simulink model "udpConnector"  (R2018b)
settings: Solver=VariableStepAuto  StartTime=0.0  StopTime=1000  RelTol=1e-3
undefined symbols (not defined in the file): f
libraries: instrumentlib x2
settings Model: Creator=root  LastModifiedBy=yuto

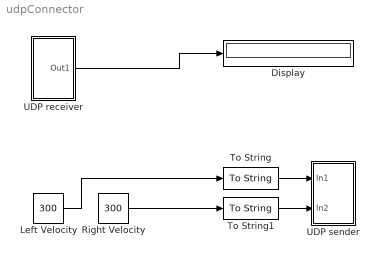
== system udpConnector ==
  Display : Display
  "Left Velocity " : Constant  Value=300
  Right Velocity : Constant  Value=300
  To String : ToString
  To String1 : ToString
  UDP receiver : Subsystem
  "UDP sender " : Subsystem
  wires:
  "Left Velocity "/1 -> To String/1
  UDP receiver/1(Out1) -> Display/1
  To String/1 -> "UDP sender "/1(In1)
  To String1/1 -> "UDP sender "/2(In2)
  Right Velocity/1 -> To String1/1

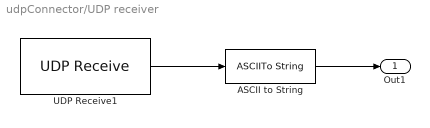
== system udpConnector/UDP receiver ==
  ASCII to String : ASCIIToString
  UDP Receive1 : instrumentlib/UDP Receive  Host=localhost  Port=9090  LocalPort=50002  EnablePortSharing=off  GetLatestData=off  DataSize="[23   1]"  DataType=uint8  ASCIIFormatting=%f,  Terminator=LF  ByteOrder=BigEndian  EnableBlockingMode=on  Timeout=10  SampleTime=0.01  LocalAddress=localhost
      settings: SourceProductName=Instrument Control Toolbox
  Out1 : Outport
  wires:
  UDP Receive1/1 -> ASCII to String/1
  ASCII to String/1 -> Out1/1

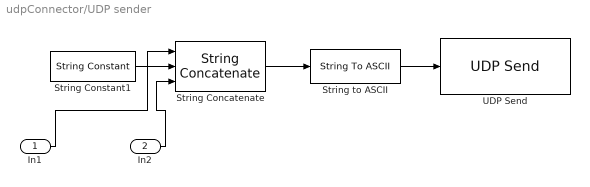
== system udpConnector/UDP sender  ==
  In1 : Inport
  In2 : Inport  Port=2
  String Concatenate : StringConcatenate  Inputs=3
  String Constant1 : StringConstant  String="\",\""
  String to ASCII : StringToASCII
  UDP Send : instrumentlib/UDP Send  Host=localhost  Port=50003  LocalPort=-1  EnablePortSharing=off  ByteOrder=BigEndian  OutputDatagramPacketSize=512  EnableBlockingMode=on  LocalAddress=0.0.0.0
      settings: SourceProductName=Instrument Control Toolbox
  wires:
  In2/1 -> String Concatenate/3
  In1/1 -> String Concatenate/1
  String Concatenate/1 -> String to ASCII/1
  String to ASCII/1 -> UDP Send/1
  String Constant1/1 -> String Concatenate/2
